simulink model "mfordmodel_v1"  (R2023a)
settings: Solver=ode45  StartTime=0.0  StopTime=10.0  RelTol=1e-3  EnableMultiTasking=on
undefined symbols (not defined in the file): ABV_RATIO_SW, AC_OFF_DLY, ACLOD, AUTO_TRNS_SW, BRAKE_DNDT_X, BZZRPM, BZZRPM_ALT, BZZTM, BZZTM_ALT, CMD_LITOFF, CMD_STABLE, CO_ST_ECT__A, COOL_BASE, DAS_BKDLY_A, DAS_CNT, DAS_CTDLY, DAS_LC_SW__A, DASCLP_5INH, DASCTL, DASMHYST, DASMPH, DEBYCP, DES_BASE, DPNEU_MUL, DSDRPM_DN_TC, DSDRPM_OFF, DSDRPM_UP_TC, EDF_DELAY, EDFHP, ETC_CL_TP, ETC_HP, GR_CM_CREEP, HCAM_ACT_CLP, HEDFHP, HEDFRPM, HICAM_PS, IAC_CAL_SW, IAC_ER_TM1, IAC_ER_TM2, IAC_ER_TM4, IAC_HI_LIM__A, IAC_ISFL_OBD, IAC_KAM_SW, IAC_LO_LIM__A, IAC_MON_TM, IAC_OT_REQ, IAC_RUN_TM, IAC_TP_OBD, IAC_TR_DAS, IAC_TST_DC, ID_DAS__A, ID_NOVS__A, IDVS_CH__A, IDVS_SL__A, IPSI_SW, IPSIDLY, IS_DRBASE__A, IS_DRBASE_A__A, IS_NUBASE__A, IS_NUBASE_A__A ... (+35)
libraries: simulink x2
(part 4 of 12)

== system mfordmodel_v1/iac_v04_001_001/iac_executive/mode_control/external_override_mode ==
  trig_external_override_mode : Inport
  osm_eo_off : Inport  Port=2
  osm_eo_on : Inport  Port=3
  osc_ena_0 : Inport  Port=4
  osc_state : Inport  Port=5
  abv_flowrate_in : Inport  Port=6
  abv_ratio_in : Inport  Port=7
  external_override_mode_ctl : Stateflow chart  TreatAsAtomicUnit=on
  flowrate_set : Subsystem  TreatAsAtomicUnit=on  mask(flowrate_set){}
      mask help: TBD
      mask Display:
      | disp('\n
      | IF (ml_flow_sel_sw == 1) THEN           \n
      |  substitute(0, abv_flowrate)\n
      | abv_ratio = 0.0                   \n
      | ELSE IF (ml_flow_sel_sw == 2) THEN\n
      | abv_flowrate = 15.99976    \n
      | abv_ratio = 0.0                    \n
      | ELSE IF (ml_flow_sel_sw == 3) THEN\n
      | abv_flowrate = 0.0              \n
      | abv_ratio = 0.0                   \n
      | ELSE IF (ml_flow_sel_sw == 4) THEN\n
      |     Do Nothing;                      \n
      | ENDIF                                                ')
  substitute : Subsystem  TreatAsAtomicUnit=on  mask(substitute){channel=0}
      mask prompts: channel "Select OSC channel"
      mask help: This block will perform Output State Control (OSC) substitution, for now it is strictly a pass-through block.
      mask TypeOptions channel: 0 | 1 | 2 | 3 | 4 | 5 | 6 | 7 | 8 | 9 | 10 | 11 | 12 | 15 | 16 | 17 | 18 | 19 | 20 | 21 | 22 | 23 | 24 | 25 | 26 | 27 | 28 | 29 | 30 | 31 | 32 | 33 | 34 | 35 | 36 | 37 | 38 | 39 | 40 | 41 | 42 | 43 | 44 | 45 | 46 | 47 | 48 | 49 | 50
      mask Display: fprintf('\nChannel # = %s\n',channel);
  abv_flowrate : Outport
  abv_ratio : Outport  Port=2
  wires:
  abv_ratio_in/1 -> flowrate_set/4(abv_ratio_in)
  flowrate_set/2(abv_ratio) -> abv_ratio/1
  flowrate_set/1(abv_flowrate) -> abv_flowrate/1
  abv_flowrate_in/1 -> flowrate_set/3(abv_flowrate_in), substitute/1(OSC_in)
  substitute/1(OSC_out) -> flowrate_set/2(abv_flowrate_osc)  "abv_flowrate_osc"
  external_override_mode_ctl/2(do_flowrate_set()) -> flowrate_set/Trigger  "do_flowrate_set"
  external_override_mode_ctl/1(ml_flow_sel_sw) -> flowrate_set/1(ml_flow_sel_sw)  "ml_flow_sel_sw"
  external_override_mode_ctl/3(do_substitute()) -> substitute/Trigger  "do_substitute"
  osc_ena_0/1 -> external_override_mode_ctl/3(osc_ena_0)
  osc_state/1 -> external_override_mode_ctl/4(osc_state)
  osm_eo_off/1 -> external_override_mode_ctl/1(osm_eo_off)
  osm_eo_on/1 -> external_override_mode_ctl/2(osm_eo_on)
  trig_external_override_mode/1 -> external_override_mode_ctl/Trigger

== system mfordmodel_v1/iac_v04_001_001/iac_executive/mode_control/failure_mode ==
  do_failure_mode : TriggerPort  TriggerType=function-call  VariantControl=(inherit)
  CONSTANT1 : Subsystem  mask(Constant){constant=IAC_FM_PPM}
      mask help: Constant Block. Will dispaly constant name and value on the icon of the block
      mask init:
      | if isletter(constant(1))
      |   const = evalin('base',constant);
      |   name = constant;
      | else
      |   const = str2num(constant);
      |   name = 'CONST';
      | end;
      mask Display: fprintf('%s = %.4f',name,const);
  Constant1 : Constant  Value=0
  Constant2 : Constant
  ISCFLG_DASHPOT_PREPOSITION : Constant  Value=0
  abv_flowrate : Outport  InitialOutput=[0]
  abv_ratio : Outport  Port=2  InitialOutput=[0]
  hcamfg : Outport  Port=3  InitialOutput=[0]
  iscflg : Outport  Port=4  InitialOutput=[0]
  wires:
  ISCFLG_DASHPOT_PREPOSITION/1 -> iscflg/1  "iscflg"
  CONSTANT1/1(Out) -> abv_flowrate/1  "abv_flowrate"
  Constant1/1 -> abv_ratio/1  "abv_ratio"
  Constant2/1 -> hcamfg/1  "hcamfg"

== system mfordmodel_v1/iac_v04_001_001/iac_executive/runup_flag_timer/TIMER_DT_in ==
  note: timer14/TIMER
  note: Timer Control calls functions within the Time Calculator
      | after using the flags 'increment_flag' and 'decrement_flag'
      | to determine the direction of the timer.
  trig_time : Inport
  trig_reset : Inport  Port=2
  reset value : Inport  Port=3
  inc flag : Inport  Port=4
  dec flag : Inport  Port=5
  delta time : Inport  Port=6
  Event Triggers : Mux  Inputs=2
  Time Calculator : Subsystem
  Timer Control : Stateflow chart  TreatAsAtomicUnit=on
  timer : Outport
  wires:
  inc flag/1 -> Timer Control/1(incr_flag)  "increment_flag"
  dec flag/1 -> Timer Control/2(decr_flag)  "decrement_flag"
  Timer Control/4(do_timer()) -> Time Calculator/4(do_timer)  "do_timer"
  Timer Control/3(do_delta_time()) -> Time Calculator/3(do_delta_time)  "do_delta_time"
  Timer Control/2(reset_flag) -> Time Calculator/2(reset_val)  "reset_flag"
  Timer Control/1(count_direction) -> Time Calculator/1(count_direction)  "count_direction"
  Time Calculator/1(timer) -> timer/1  "timer"
  Event Triggers/1 -> Timer Control/Trigger
  trig_time/1 -> Event Triggers/1  "trig_timer"
  trig_reset/1 -> Event Triggers/2  "trig_reset"
  reset value/1 -> Time Calculator/5(reset_value)  "reset_value"
  delta time/1 -> Time Calculator/6(delta time)  "delta_time"

== system mfordmodel_v1/iac_v04_001_001/normal_mode/activate_feedforward/ac_ppm_tmr ==
  note: Timer Control calls functions within the Time Calculator
      | after using the flags 'increment_flag' and 'decrement_flag'
      | to determine the direction of the timer.
  note: timer14/TIMER
  trig_time : Inport
  trig_reset : Inport  Port=2
  reset value : Inport  Port=3
  inc flag : Inport  Port=4
  dec flag : Inport  Port=5
  Event Triggers : Mux  Inputs=2
  Time Calculator : Subsystem
  Timer Control : Stateflow chart  TreatAsAtomicUnit=on
  timer : Outport
  wires:
  reset value/1 -> Time Calculator/5(reset_value)  "reset_value"
  trig_reset/1 -> Event Triggers/2  "trig_reset"
  trig_time/1 -> Event Triggers/1  "trig_timer"
  Event Triggers/1 -> Timer Control/Trigger
  Time Calculator/1(timer) -> timer/1  "timer"
  Timer Control/1(count_direction) -> Time Calculator/1(count_direction)  "count_direction"
  Timer Control/2(reset_flag) -> Time Calculator/2(reset_val)  "reset_flag"
  Timer Control/3(do_delta_time()) -> Time Calculator/3(do_delta_time)  "do_delta_time"
  Timer Control/4(do_timer()) -> Time Calculator/4(do_timer)  "do_timer"
  dec flag/1 -> Timer Control/2(decr_flag)  "decrement_flag"
  inc flag/1 -> Timer Control/1(incr_flag)  "increment_flag"

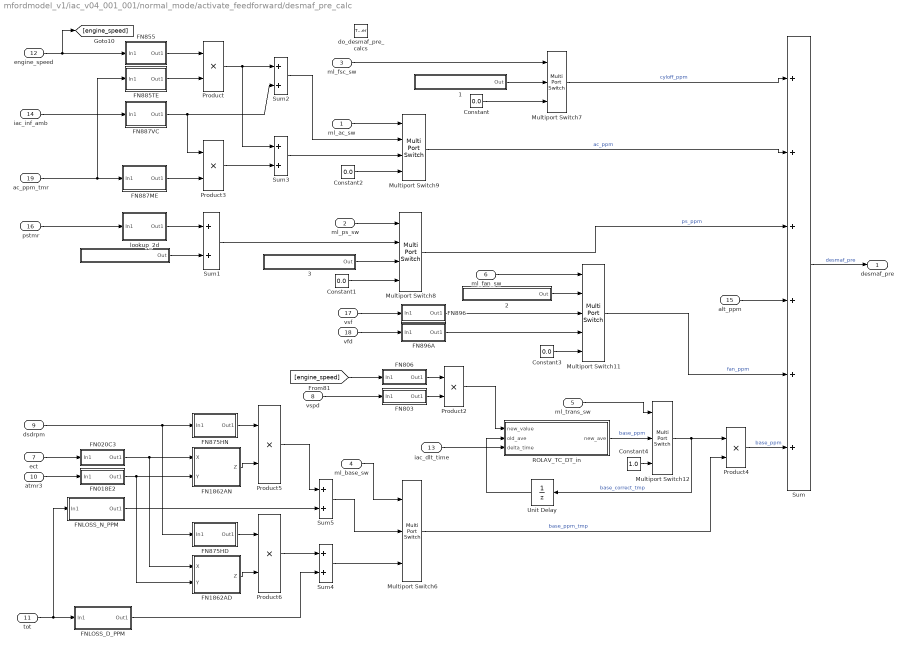
== system mfordmodel_v1/iac_v04_001_001/normal_mode/activate_feedforward/desmaf_pre_calc ==
  ml_ac_sw : Inport
  ml_ps_sw : Inport  Port=2
  ml_fsc_sw : Inport  Port=3
  ml_base_sw : Inport  Port=4
  ml_trans_sw : Inport  Port=5
  ml_fan_sw : Inport  Port=6
  ect : Inport  Port=7
  vspd : Inport  Port=8
  dsdrpm : Inport  Port=9
  atmr3 : Inport  Port=10
  tot : Inport  Port=11
  engine_speed : Inport  Port=12
  iac_dlt_time : Inport  Port=13
  iac_inf_amb : Inport  Port=14
  alt_ppm : Inport  Port=15
  pstmr : Inport  Port=16
  vsf : Inport  Port=17
  vfd : Inport  Port=18
  ac_ppm_tmr : Inport  Port=19
  do_desmaf_pre_calcs : TriggerPort  TriggerType=function-call  VariantControl=(inherit)
  "  " : Subsystem  mask(Constant){constant=PSPPM}
      mask help: Constant Block. Will dispaly constant name and value on the icon of the block
      mask init:
      | if isletter(constant(1))
      |   const = evalin('base',constant);
      |   name = constant;
      | else
      |   const = str2num(constant);
      |   name = 'CONST';
      | end;
      mask Display: fprintf('%s = %.4f',name,const);
  "  2" : Subsystem  mask(Constant){constant=EDFPPM}
      mask help: Constant Block. Will dispaly constant name and value on the icon of the block
      mask init:
      | if isletter(constant(1))
      |   const = evalin('base',constant);
      |   name = constant;
      | else
      |   const = str2num(constant);
      |   name = 'CONST';
      | end;
      mask Display: fprintf('%s = %.4f',name,const);
  1 : Subsystem  mask(Constant){constant=FSC_BASE_PPM}
      mask help: Constant Block. Will dispaly constant name and value on the icon of the block
      mask init:
      | if isletter(constant(1))
      |   const = evalin('base',constant);
      |   name = constant;
      | else
      |   const = str2num(constant);
      |   name = 'CONST';
      | end;
      mask Display: fprintf('%s = %.4f',name,const);
  3 : Subsystem  mask(Constant){constant=PSPPM_VS}
      mask help: Constant Block. Will dispaly constant name and value on the icon of the block
      mask init:
      | if isletter(constant(1))
      |   const = evalin('base',constant);
      |   name = constant;
      | else
      |   const = str2num(constant);
      |   name = 'CONST';
      | end;
      mask Display: fprintf('%s = %.4f',name,const);
  Constant{,1..3} (4 alike) : Constant  Value=0.0
  Constant4 : Constant  Value=1.0
  FN018E2 : Subsystem  mask(2-D, piece-wise, linear interpolation){CAL_FUNC=FN018E}
      mask prompts: CAL_FUNC "Calibration function name"
      mask help:
      | Performs piece-wise linear interpolation.
      |
      | Output is NOT extrapolated beyond the input range.  If the input value presented to the block lies outside the range specified in the block's parameter, then the value is treated as though it has the value of the nearest value in the range.
      mask init: same as mfordmodel_v1/iac_v04_001_001/activate_desired_rpm/rpm_calcs/lookup_2d
      mask Help:
      | Enter the name of the calibration function.
      | (e.g. EGM_VA_ECT_MULT)
      mask Display:
      | fprintf('%s',CAL_FUNC);
      | plot(calfunc.X,calfunc.Y,max_x*1.05,max_y*1.05,min_x,min_y);
  FN020C3 : Subsystem  mask(2-D, piece-wise, linear interpolation){CAL_FUNC=FN020C}
      mask prompts: CAL_FUNC "Calibration function name"
      mask help:
      | Performs piece-wise linear interpolation.
      |
      | Output is NOT extrapolated beyond the input range.  If the input value presented to the block lies outside the range specified in the block's parameter, then the value is treated as though it has the value of the nearest value in the range.
      mask init: same as mfordmodel_v1/iac_v04_001_001/activate_desired_rpm/rpm_calcs/lookup_2d
      mask Help:
      | Enter the name of the calibration function.
      | (e.g. EGM_VA_ECT_MULT)
      mask Display:
      | fprintf('%s',CAL_FUNC);
      | plot(calfunc.X,calfunc.Y,max_x*1.05,max_y*1.05,min_x,min_y);
  FN1862AD : Subsystem  mask(3-D, piece-wise, linear interpolation){CAL_TABLE=FN1862AD}
      mask prompts: CAL_TABLE "Calibration table name"
      mask help:
      | Performs 3-D, piece-wise linear interpolation.
      |
      | Output is NOT extrapolated beyond the input ranges.  If an input value presented to the block lies outside the range specified in the block's parameters, then the value is treated as though it has the value of the nearest value in the range.
      mask init:
      | if isempty(CAL_TABLE) |  isspace(CAL_TABLE)
      |  caltable.Z=[0 .05 .1 .1 ;.1 .15 .2 .2; .2 .25 .3 .3;.3 .35 .4 .4];
      |  min_x=0;
      |  min_y=0;
      |  max_x=3;
      |  max_y=3;
      |  minz=0;
      |  maxz=1;
      |  CAL_TABLE='FNxxxx';
      | else
      |   caltable = evalin('base',CAL_TABLE);
      |   min_x = caltable.X(1);
      |   max_x = caltable.X(length(caltable.X));
      |   min_y = caltable.Y(1);
      |   max_y = caltable.Y(length(caltable.Y));
      |   minz=min(min(caltable.Z));
      |   maxz=max(max(caltable.Z));
      | end
      mask Help: Enter the name of the calibration table.
      mask Display:
      | fprintf('%s',CAL_TABLE);
      | plot(caltable.Z');
      | plot([min_x max_x],[minz*.99 minz*.99]);
      | plot([min_x min_x],[minz*.99 maxz*1.01]);
  FN1862AN : Subsystem  mask(3-D, piece-wise, linear interpolation){CAL_TABLE=FN1862AN}
      mask prompts: CAL_TABLE "Calibration table name"
      mask help:
      | Performs 3-D, piece-wise linear interpolation.
      |
      | Output is NOT extrapolated beyond the input ranges.  If an input value presented to the block lies outside the range specified in the block's parameters, then the value is treated as though it has the value of the nearest value in the range.
      mask init: same as mfordmodel_v1/iac_v04_001_001/normal_mode/activate_feedforward/desmaf_pre_calc/FN1862AD
      mask Help: Enter the name of the calibration table.
      mask Display:
      | fprintf('%s',CAL_TABLE);
      | plot(caltable.Z');
      | plot([min_x max_x],[minz*.99 minz*.99]);
      | plot([min_x min_x],[minz*.99 maxz*1.01]);
  FN803 : Subsystem  mask(2-D, piece-wise, linear interpolation){CAL_FUNC=FN802}
      mask prompts: CAL_FUNC "Calibration function name"
      mask help:
      | Performs piece-wise linear interpolation.
      |
      | Output is NOT extrapolated beyond the input range.  If the input value presented to the block lies outside the range specified in the block's parameter, then the value is treated as though it has the value of the nearest value in the range.
      mask init: same as mfordmodel_v1/iac_v04_001_001/activate_desired_rpm/rpm_calcs/lookup_2d
      mask Help:
      | Enter the name of the calibration function.
      | (e.g. EGM_VA_ECT_MULT)
      mask Display:
      | fprintf('%s',CAL_FUNC);
      | plot(calfunc.X,calfunc.Y,max_x*1.05,max_y*1.05,min_x,min_y);
  FN806 : Subsystem  mask(2-D, piece-wise, linear interpolation){CAL_FUNC=FN805}
      mask prompts: CAL_FUNC "Calibration function name"
      mask help:
      | Performs piece-wise linear interpolation.
      |
      | Output is NOT extrapolated beyond the input range.  If the input value presented to the block lies outside the range specified in the block's parameter, then the value is treated as though it has the value of the nearest value in the range.
      mask init: same as mfordmodel_v1/iac_v04_001_001/activate_desired_rpm/rpm_calcs/lookup_2d
      mask Help:
      | Enter the name of the calibration function.
      | (e.g. EGM_VA_ECT_MULT)
      mask Display:
      | fprintf('%s',CAL_FUNC);
      | plot(calfunc.X,calfunc.Y,max_x*1.05,max_y*1.05,min_x,min_y);
  FN855 : Subsystem  mask(2-D, piece-wise, linear interpolation){CAL_FUNC=FN885}
      mask prompts: CAL_FUNC "Calibration function name"
      mask help:
      | Performs piece-wise linear interpolation.
      |
      | Output is NOT extrapolated beyond the input range.  If the input value presented to the block lies outside the range specified in the block's parameter, then the value is treated as though it has the value of the nearest value in the range.
      mask init: same as mfordmodel_v1/iac_v04_001_001/activate_desired_rpm/rpm_calcs/lookup_2d
      mask Help:
      | Enter the name of the calibration function.
      | (e.g. EGM_VA_ECT_MULT)
      mask Display:
      | fprintf('%s',CAL_FUNC);
      | plot(calfunc.X,calfunc.Y,max_x*1.05,max_y*1.05,min_x,min_y);
  FN875HD : Subsystem  mask(2-D, piece-wise, linear interpolation){CAL_FUNC=FN875HD}
      mask prompts: CAL_FUNC "Calibration function name"
      mask help:
      | Performs piece-wise linear interpolation.
      |
      | Output is NOT extrapolated beyond the input range.  If the input value presented to the block lies outside the range specified in the block's parameter, then the value is treated as though it has the value of the nearest value in the range.
      mask init: same as mfordmodel_v1/iac_v04_001_001/activate_desired_rpm/rpm_calcs/lookup_2d
      mask Help:
      | Enter the name of the calibration function.
      | (e.g. EGM_VA_ECT_MULT)
      mask Display:
      | fprintf('%s',CAL_FUNC);
      | plot(calfunc.X,calfunc.Y,max_x*1.05,max_y*1.05,min_x,min_y);
  FN875HN : Subsystem  mask(2-D, piece-wise, linear interpolation){CAL_FUNC=FN875HN}
      mask prompts: CAL_FUNC "Calibration function name"
      mask help:
      | Performs piece-wise linear interpolation.
      |
      | Output is NOT extrapolated beyond the input range.  If the input value presented to the block lies outside the range specified in the block's parameter, then the value is treated as though it has the value of the nearest value in the range.
      mask init: same as mfordmodel_v1/iac_v04_001_001/activate_desired_rpm/rpm_calcs/lookup_2d
      mask Help:
      | Enter the name of the calibration function.
      | (e.g. EGM_VA_ECT_MULT)
      mask Display:
      | fprintf('%s',CAL_FUNC);
      | plot(calfunc.X,calfunc.Y,max_x*1.05,max_y*1.05,min_x,min_y);
  FN885TE : Subsystem  mask(2-D, piece-wise, linear interpolation){CAL_FUNC=FN885TE}
      mask prompts: CAL_FUNC "Calibration function name"
      mask help:
      | Performs piece-wise linear interpolation.
      |
      | Output is NOT extrapolated beyond the input range.  If the input value presented to the block lies outside the range specified in the block's parameter, then the value is treated as though it has the value of the nearest value in the range.
      mask init: same as mfordmodel_v1/iac_v04_001_001/activate_desired_rpm/rpm_calcs/lookup_2d
      mask Help:
      | Enter the name of the calibration function.
      | (e.g. EGM_VA_ECT_MULT)
      mask Display:
      | fprintf('%s',CAL_FUNC);
      | plot(calfunc.X,calfunc.Y,max_x*1.05,max_y*1.05,min_x,min_y);
  FN887ME : Subsystem  mask(2-D, piece-wise, linear interpolation){CAL_FUNC=FN887ME}
      mask prompts: CAL_FUNC "Calibration function name"
      mask help:
      | Performs piece-wise linear interpolation.
      |
      | Output is NOT extrapolated beyond the input range.  If the input value presented to the block lies outside the range specified in the block's parameter, then the value is treated as though it has the value of the nearest value in the range.
      mask init: same as mfordmodel_v1/iac_v04_001_001/activate_desired_rpm/rpm_calcs/lookup_2d
      mask Help:
      | Enter the name of the calibration function.
      | (e.g. EGM_VA_ECT_MULT)
      mask Display:
      | fprintf('%s',CAL_FUNC);
      | plot(calfunc.X,calfunc.Y,max_x*1.05,max_y*1.05,min_x,min_y);
  FN887VC : Subsystem  mask(2-D, piece-wise, linear interpolation){CAL_FUNC=FN887VC}
      mask prompts: CAL_FUNC "Calibration function name"
      mask help:
      | Performs piece-wise linear interpolation.
      |
      | Output is NOT extrapolated beyond the input range.  If the input value presented to the block lies outside the range specified in the block's parameter, then the value is treated as though it has the value of the nearest value in the range.
      mask init: same as mfordmodel_v1/iac_v04_001_001/activate_desired_rpm/rpm_calcs/lookup_2d
      mask Help:
      | Enter the name of the calibration function.
      | (e.g. EGM_VA_ECT_MULT)
      mask Display:
      | fprintf('%s',CAL_FUNC);
      | plot(calfunc.X,calfunc.Y,max_x*1.05,max_y*1.05,min_x,min_y);
  FN896 : Subsystem  mask(2-D, piece-wise, linear interpolation){CAL_FUNC=FN896}
      mask prompts: CAL_FUNC "Calibration function name"
      mask help:
      | Performs piece-wise linear interpolation.
      |
      | Output is NOT extrapolated beyond the input range.  If the input value presented to the block lies outside the range specified in the block's parameter, then the value is treated as though it has the value of the nearest value in the range.
      mask init: same as mfordmodel_v1/iac_v04_001_001/activate_desired_rpm/rpm_calcs/lookup_2d
      mask Help:
      | Enter the name of the calibration function.
      | (e.g. EGM_VA_ECT_MULT)
      mask Display:
      | fprintf('%s',CAL_FUNC);
      | plot(calfunc.X,calfunc.Y,max_x*1.05,max_y*1.05,min_x,min_y);
  FN896A : Subsystem  mask(2-D, piece-wise, linear interpolation){CAL_FUNC=FN896A}
      mask prompts: CAL_FUNC "Calibration function name"
      mask help:
      | Performs piece-wise linear interpolation.
      |
      | Output is NOT extrapolated beyond the input range.  If the input value presented to the block lies outside the range specified in the block's parameter, then the value is treated as though it has the value of the nearest value in the range.
      mask init: same as mfordmodel_v1/iac_v04_001_001/activate_desired_rpm/rpm_calcs/lookup_2d
      mask Help:
      | Enter the name of the calibration function.
      | (e.g. EGM_VA_ECT_MULT)
      mask Display:
      | fprintf('%s',CAL_FUNC);
      | plot(calfunc.X,calfunc.Y,max_x*1.05,max_y*1.05,min_x,min_y);
  FNLOSS_D_PPM : Subsystem  mask(2-D, piece-wise, linear interpolation){CAL_FUNC=FNLOSS_D_PPM}
      mask prompts: CAL_FUNC "Calibration function name"
      mask help:
      | Performs piece-wise linear interpolation.
      |
      | Output is NOT extrapolated beyond the input range.  If the input value presented to the block lies outside the range specified in the block's parameter, then the value is treated as though it has the value of the nearest value in the range.
      mask init: same as mfordmodel_v1/iac_v04_001_001/activate_desired_rpm/rpm_calcs/lookup_2d
      mask Help:
      | Enter the name of the calibration function.
      | (e.g. EGM_VA_ECT_MULT)
      mask Display:
      | fprintf('%s',CAL_FUNC);
      | plot(calfunc.X,calfunc.Y,max_x*1.05,max_y*1.05,min_x,min_y);
  FNLOSS_N_PPM : Subsystem  mask(2-D, piece-wise, linear interpolation){CAL_FUNC=FNLOSS_N_PPM}
      mask prompts: CAL_FUNC "Calibration function name"
      mask help:
      | Performs piece-wise linear interpolation.
      |
      | Output is NOT extrapolated beyond the input range.  If the input value presented to the block lies outside the range specified in the block's parameter, then the value is treated as though it has the value of the nearest value in the range.
      mask init: same as mfordmodel_v1/iac_v04_001_001/activate_desired_rpm/rpm_calcs/lookup_2d
      mask Help:
      | Enter the name of the calibration function.
      | (e.g. EGM_VA_ECT_MULT)
      mask Display:
      | fprintf('%s',CAL_FUNC);
      | plot(calfunc.X,calfunc.Y,max_x*1.05,max_y*1.05,min_x,min_y);
  Multiport Switch11 : MultiPortSwitch  Inputs=4
  Multiport Switch12 : MultiPortSwitch  Inputs=2
  Multiport Switch6 : MultiPortSwitch  Inputs=2
  Multiport Switch7 : MultiPortSwitch  Inputs=2
  Multiport Switch8 : MultiPortSwitch
  Multiport Switch9 : MultiPortSwitch
  Product{,2..6} (6 alike) : Product  InputSameDT=on  RndMeth=Zero  SaturateOnIntegerOverflow=on  OutDataTypeStr=Inherit: Same as first input
  ROLAV_TC_DT_in : Subsystem  mask(Rolling Average - Time Constant){TAU=TCDAIR}
      mask prompts: TAU "Time Constant"
      mask help: Rolling Average - Time Constant. This filter block is the first order approximation using a time constant. Inputs include the time constant (entered through this dialogue), old_ave which is the previous average value, new_value which is the new filter to filter toward, and the delta_time which is elapsed time over which to perform the filter equation.
      mask init:
      | if isletter(TAU(1))
      |   tc = evalin('base',TAU);
      |   name = TAU;
      | else
      |   tc = str2num(TAU);
      |   name = 'TC';
      | end;
      mask Display: fprintf('%s = %.4f',name,tc);
  Sum : Sum  Inputs=++++++  InputSameDT=on  SaturateOnIntegerOverflow=on  OutDataTypeStr=Inherit: Same as first input
  Sum{1..5} (5 alike) : Sum  InputSameDT=on  SaturateOnIntegerOverflow=on  OutDataTypeStr=Inherit: Same as first input
  Unit Delay : UnitDelay  InitialCondition=1.0  SampleTime=-1
  lookup_2d : Subsystem  mask(2-D, piece-wise, linear interpolation){CAL_FUNC=FN822}
      mask prompts: CAL_FUNC "Calibration function name"
      mask help:
      | Performs piece-wise linear interpolation.
      |
      | Output is NOT extrapolated beyond the input range.  If the input value presented to the block lies outside the range specified in the block's parameter, then the value is treated as though it has the value of the nearest value in the range.
      mask init: same as mfordmodel_v1/iac_v04_001_001/activate_desired_rpm/rpm_calcs/lookup_2d
      mask Help:
      | Enter the name of the calibration function.
      | (e.g. EGM_VA_ECT_MULT)
      mask Display:
      | fprintf('%s',CAL_FUNC);
      | plot(calfunc.X,calfunc.Y,max_x*1.05,max_y*1.05,min_x,min_y);
  desmaf_pre : Outport
  wires:
  FN803/1(Out1) -> Product2/2
  FN806/1(Out1) -> Product2/1
  vspd/1 -> FN803/1(In1)
  [engine_speed] -> FN806/1(In1)
  Unit Delay/1 -> ROLAV_TC_DT_in/2(old_ave)
  Product2/1 -> ROLAV_TC_DT_in/1(new_value)
  iac_dlt_time/1 -> ROLAV_TC_DT_in/3(delta_time)
  Constant3/1 -> Multiport Switch11/5
  vfd/1 -> FN896A/1(In1)
  vsf/1 -> FN896/1(In1)
  FN896/1(Out1) -> Multiport Switch11/3
  Multiport Switch11/1 -> Sum/5  "fan_ppm"
  FN896A/1(Out1) -> Multiport Switch11/4
  "  2"/1(Out) -> Multiport Switch11/2
  ml_fan_sw/1 -> Multiport Switch11/1
  Multiport Switch12/1 -> Unit Delay/1, Product4/1  "base_correct_tmp"
  ROLAV_TC_DT_in/1(new_ave) -> Multiport Switch12/2  "base_ppm"
  ml_trans_sw/1 -> Multiport Switch12/1
  Constant4/1 -> Multiport Switch12/3
  Multiport Switch6/1 -> Product4/2  "base_ppm_tmp"
  FN875HN/1(Out1) -> Product5/1
  FN1862AN/1(Z) -> Product5/2
  ml_base_sw/1 -> Multiport Switch6/1
  atmr3/1 -> FN018E2/1(In1)
  FN020C3/1(Out1) -> FN1862AN/1(X), FN1862AD/1(X)
  FN018E2/1(Out1) -> FN1862AN/2(Y), FN1862AD/2(Y)
  ect/1 -> FN020C3/1(In1)
  dsdrpm/1 -> FN875HN/1(In1), FN875HD/1(In1)
  Product5/1 -> Sum5/1
  FNLOSS_N_PPM/1(Out1) -> Sum5/2
  Sum5/1 -> Multiport Switch6/2
  Product6/1 -> Sum4/1
  Sum4/1 -> Multiport Switch6/3
  FNLOSS_D_PPM/1(Out1) -> Sum4/2
  FN875HD/1(Out1) -> Product6/1
  FN1862AD/1(Z) -> Product6/2
  tot/1 -> FNLOSS_D_PPM/1(In1), FNLOSS_N_PPM/1(In1)
  Product4/1 -> Sum/6  "base_ppm"
  Sum/1 -> desmaf_pre/1  "desmaf_pre"
  FN855/1(Out1) -> Product/1
  FN885TE/1(Out1) -> Product/2
  alt_ppm/1 -> Sum/4
  Multiport Switch8/1 -> Sum/3  "ps_ppm"
  Multiport Switch9/1 -> Sum/2  "ac_ppm"
  Sum2/1 -> Multiport Switch9/2
  Sum3/1 -> Multiport Switch9/3
  Constant2/1 -> Multiport Switch9/4
  ml_ac_sw/1 -> Multiport Switch9/1
  Product3/1 -> Sum3/2
  FN887ME/1(Out1) -> Product3/2
  Product/1 -> Sum2/1, Sum3/1
  FN887VC/1(Out1) -> Sum2/2, Product3/1
  engine_speed/1 -> [engine_speed], FN855/1(In1)
  iac_inf_amb/1 -> FN887VC/1(In1)
  ac_ppm_tmr/1 -> FN887ME/1(In1), FN885TE/1(In1)
  lookup_2d/1(Out1) -> Sum1/1
  "  "/1(Out) -> Sum1/2
  Constant1/1 -> Multiport Switch8/4
  ml_ps_sw/1 -> Multiport Switch8/1
  3/1(Out) -> Multiport Switch8/3
  Sum1/1 -> Multiport Switch8/2
  pstmr/1 -> lookup_2d/1(In1)
  Multiport Switch7/1 -> Sum/1  "cyloff_ppm"
  Constant/1 -> Multiport Switch7/3
  1/1(Out) -> Multiport Switch7/2
  ml_fsc_sw/1 -> Multiport Switch7/1

== system mfordmodel_v1/iac_v04_001_001/normal_mode/activate_kam/iac_kam_tmr ==
  note: Timer Control calls functions within the Time Calculator
      | after using the flags 'increment_flag' and 'decrement_flag'
      | to determine the direction of the timer.
  note: timer14/TIMER
  trig_time : Inport
  trig_reset : Inport  Port=2
  reset value : Inport  Port=3
  inc flag : Inport  Port=4
  dec flag : Inport  Port=5
  Event Triggers : Mux  Inputs=2
  Time Calculator : Subsystem
  Timer Control : Stateflow chart  TreatAsAtomicUnit=on
  timer : Outport
  wires:
  reset value/1 -> Time Calculator/5(reset_value)  "reset_value"
  trig_reset/1 -> Event Triggers/2  "trig_reset"
  trig_time/1 -> Event Triggers/1  "trig_timer"
  Event Triggers/1 -> Timer Control/Trigger
  Time Calculator/1(timer) -> timer/1  "timer"
  Timer Control/1(count_direction) -> Time Calculator/1(count_direction)  "count_direction"
  Timer Control/2(reset_flag) -> Time Calculator/2(reset_val)  "reset_flag"
  Timer Control/3(do_delta_time()) -> Time Calculator/3(do_delta_time)  "do_delta_time"
  Timer Control/4(do_timer()) -> Time Calculator/4(do_timer)  "do_timer"
  dec flag/1 -> Timer Control/2(decr_flag)  "decrement_flag"
  inc flag/1 -> Timer Control/1(incr_flag)  "increment_flag"

== system mfordmodel_v1/iac_v04_001_001/normal_mode/activate_kam/isckam_calcs ==
  ipsibr_fb : Inport
  ml_kam_inc_sw : Inport  Port=2
  ml_isflag_sw : Inport  Port=3
  isckam_in : Inport  Port=4
  iac_ac_n_kam_in : Inport  Port=5
  iac_ac_d_kam_in : Inport  Port=6
  do_isckam_calcs : TriggerPort  TriggerType=function-call  VariantControl=(inherit)
  Bus Selector2 : BusSelector  OutputSignals=isckam0
  Bus Selector3 : BusSelector  OutputSignals=isckam2
  Constant1 : Constant  Value=0.0
  Constant7 : Constant  Value=.0003
  Constant8 : Constant  Value=-.0003
  Multiport Switch{17..18,24..25} (4 alike) : MultiPortSwitch  Inputs=4
  Multiport Switch23 : MultiPortSwitch
  Mux : Mux
  Sum{10..13} (4 alike) : Sum  Inputs=|++  InputSameDT=on  SaturateOnIntegerOverflow=on  OutDataTypeStr=Inherit: Same as first input
  Sum15 : Sum  Inputs=+-  InputSameDT=on  SaturateOnIntegerOverflow=on  OutDataTypeStr=Inherit: Same as first input
  Sum16 : Sum  InputSameDT=on  SaturateOnIntegerOverflow=on  OutDataTypeStr=Inherit: Same as first input
  Sum18 : Sum  InputSameDT=on  SaturateOnIntegerOverflow=on  OutDataTypeStr=Inherit: Same as first input
  ipsibr_kam : Outport
  isckam : Outport  Port=2
  iac_ac_n_kam : Outport  Port=3
  iac_ac_d_kam : Outport  Port=4
  wires:
  ml_kam_inc_sw/1 -> Multiport Switch23/1
  Constant1/1 -> Multiport Switch23/4
  Constant8/1 -> Multiport Switch23/2
  Constant7/1 -> Multiport Switch23/3
  Multiport Switch23/1 -> [increment_tmp], Sum15/2  "increment_tmp"
  Mux/1 -> isckam/1  "ml_isckam"
  Sum16/1 -> Mux/2  "isckam1"
  Sum18/1 -> Mux/4  "isckam3"
  [ml_isflag_sw] -> Multiport Switch18/1
  Sum11/1 -> Multiport Switch18/4
  [increment_tmp] -> Sum11/1
  Sum10/1 -> Multiport Switch17/5
  [ml_isflag_sw] -> Multiport Switch17/1
  [increment_tmp] -> Sum10/2
  [ml_isflag_sw] -> Multiport Switch24/1
  Sum12/1 -> Multiport Switch24/3
  [increment_tmp] -> Sum12/1
  ml_isflag_sw/1 -> [ml_isflag_sw], Multiport Switch25/1
  Sum13/1 -> Multiport Switch25/2
  [increment_tmp] -> Sum13/1
  isckam_in/1 -> Bus Selector2/1, Bus Selector3/1
  ipsibr_fb/1 -> Sum15/1
  Sum15/1 -> ipsibr_kam/1  "ipsibr_kam"
  Multiport Switch17/1 -> iac_ac_n_kam/1  "iac_ac_n_kam"
  iac_ac_n_kam_in/1 -> Multiport Switch17/2, Multiport Switch17/3, Multiport Switch17/4, Sum10/1, [iac_ac_n_kam]
  Multiport Switch24/1 -> iac_ac_d_kam/1  "iac_ac_d_kam"
  iac_ac_d_kam_in/1 -> Multiport Switch24/2, Multiport Switch24/5, Multiport Switch24/4, Sum12/2, [iac_ac_d_kam]
  Multiport Switch25/1 -> Mux/1  "isckam0"
  Multiport Switch18/1 -> Mux/3  "isckam2"
  Bus Selector2/1 -> Multiport Switch25/5, Sum13/2, Multiport Switch25/3, Multiport Switch25/4, [isckam0]  "<isckam0>"
  Bus Selector3/1 -> Multiport Switch18/2, Multiport Switch18/3, Multiport Switch18/5, Sum11/2, [isckam2]  "<isckam2>"
  [iac_ac_d_kam] -> Sum16/2
  [isckam0] -> Sum16/1
  [iac_ac_n_kam] -> Sum18/2
  [isckam2] -> Sum18/1

== system mfordmodel_v1/iac_v04_001_001/normal_mode/activate_kam/isckam_clear ==
  note: These connection is made via
      | a constant block here instead of a goto/from
      | tag because the actual signals
      | are connected to merge blocks and sumulink
      | does not allow multiple connections for
      | signal lines connected to merge blocks.
  do_isckam_clear : TriggerPort  TriggerType=function-call  VariantControl=(inherit)
  CONSTANT1 : Subsystem  mask(Constant){constant=IAC_AC_START}
      mask help: Constant Block. Will dispaly constant name and value on the icon of the block
      mask init:
      | if isletter(constant(1))
      |   const = evalin('base',constant);
      |   name = constant;
      | else
      |   const = str2num(constant);
      |   name = 'CONST';
      | end;
      mask Display: fprintf('%s = %.4f',name,const);
  CONSTANT2 : Subsystem  mask(Constant){constant=IAC_NU_START}
      mask help: Constant Block. Will dispaly constant name and value on the icon of the block
      mask init:
      | if isletter(constant(1))
      |   const = evalin('base',constant);
      |   name = constant;
      | else
      |   const = str2num(constant);
      |   name = 'CONST';
      | end;
      mask Display: fprintf('%s = %.4f',name,const);
  CONSTANT3 : Subsystem  mask(Constant){constant=IAC_DR_START}
      mask help: Constant Block. Will dispaly constant name and value on the icon of the block
      mask init:
      | if isletter(constant(1))
      |   const = evalin('base',constant);
      |   name = constant;
      | else
      |   const = str2num(constant);
      |   name = 'CONST';
      | end;
      mask Display: fprintf('%s = %.4f',name,const);
  CONSTANT4 : Subsystem  mask(Constant){constant=IAC_AC_START}
      mask help: Constant Block. Will dispaly constant name and value on the icon of the block
      mask init:
      | if isletter(constant(1))
      |   const = evalin('base',constant);
      |   name = constant;
      | else
      |   const = str2num(constant);
      |   name = 'CONST';
      | end;
      mask Display: fprintf('%s = %.4f',name,const);
  CONSTANT5 : Subsystem  mask(Constant){constant=IAC_DR_START}
      mask help: Constant Block. Will dispaly constant name and value on the icon of the block
      mask init:
      | if isletter(constant(1))
      |   const = evalin('base',constant);
      |   name = constant;
      | else
      |   const = str2num(constant);
      |   name = 'CONST';
      | end;
      mask Display: fprintf('%s = %.4f',name,const);
  CONSTANT6 : Subsystem  mask(Constant){constant=IAC_NU_START}
      mask help: Constant Block. Will dispaly constant name and value on the icon of the block
      mask init:
      | if isletter(constant(1))
      |   const = evalin('base',constant);
      |   name = constant;
      | else
      |   const = str2num(constant);
      |   name = 'CONST';
      | end;
      mask Display: fprintf('%s = %.4f',name,const);
  CONSTANT7 : Subsystem  mask(Constant){constant=IAC_AC_START}
      mask help: Constant Block. Will dispaly constant name and value on the icon of the block
      mask init:
      | if isletter(constant(1))
      |   const = evalin('base',constant);
      |   name = constant;
      | else
      |   const = str2num(constant);
      |   name = 'CONST';
      | end;
      mask Display: fprintf('%s = %.4f',name,const);
  CONSTANT8 : Subsystem  mask(Constant){constant=IAC_AC_START}
      mask help: Constant Block. Will dispaly constant name and value on the icon of the block
      mask init:
      | if isletter(constant(1))
      |   const = evalin('base',constant);
      |   name = constant;
      | else
      |   const = str2num(constant);
      |   name = 'CONST';
      | end;
      mask Display: fprintf('%s = %.4f',name,const);
  Constant : Constant  Value=0.0
  Constant1 : Constant  Value=0.0
  Mux : Mux
  Sum1 : Sum  Inputs=++++  InputSameDT=on  SaturateOnIntegerOverflow=on  OutDataTypeStr=Inherit: Same as first input
  isckam : Outport
  iac_ac_n_kam : Outport  Port=2
  iac_ac_d_kam : Outport  Port=3
  iac_chksum : Outport  Port=4
  wires:
  Mux/1 -> isckam/1  "ml_isckam"
  Constant/1 -> Mux/2  "isckam1"
  Constant1/1 -> Mux/4  "isckam3"
  CONSTANT3/1(Out) -> Mux/1  "isckam0"
  CONSTANT2/1(Out) -> Mux/3  "isckam2"
  Sum1/1 -> iac_chksum/1  "iac_chksum"
  CONSTANT5/1(Out) -> Sum1/2  "isckam0"
  CONSTANT6/1(Out) -> Sum1/1  "isckam2"
  CONSTANT7/1(Out) -> Sum1/3  "iac_ac_n_kam"
  CONSTANT8/1(Out) -> Sum1/4  "iac_ac_n_kam"
  CONSTANT1/1(Out) -> iac_ac_n_kam/1  "iac_ac_n_kam"
  CONSTANT4/1(Out) -> iac_ac_d_kam/1  "iac_ac_d_kam"

== system mfordmodel_v1/iac_v04_001_001/normal_mode/activate_kam/isckam_merge ==
  ml_isckam1 : Inport
  ml_isckam2 : Inport  Port=2
  Demux : Demux
      settings: DisplayOption=none
  Demux1 : Demux
      settings: DisplayOption=none
  Merge{3..6} (4 alike) : Merge
  Mux : Mux
  isckam : Outport
  wires:
  Demux1/4 -> Merge6/2
  Demux1/3 -> Merge5/2
  Demux1/2 -> Merge4/2
  Demux1/1 -> Merge3/2
  ml_isckam2/1 -> Demux1/1
  ml_isckam1/1 -> Demux/1
  Mux/1 -> isckam/1
  Merge6/1 -> Mux/4  "isckam3"
  Merge5/1 -> Mux/3  "isckam2"
  Merge4/1 -> Mux/2  "isckam1"
  Merge3/1 -> Mux/1  "isckam0"
  Demux/4 -> Merge6/1
  Demux/3 -> Merge5/1
  Demux/2 -> Merge4/1
  Demux/1 -> Merge3/1

== system mfordmodel_v1/iac_v04_001_001/normal_mode/activate_kam/isckam_update_checksum ==
  iac_ac_n_kam : Inport
  iac_ac_d_kam : Inport  Port=2
  isckam : Inport  Port=3
  do_isckam_update_checksum : TriggerPort  TriggerType=function-call  VariantControl=(inherit)
  Bus Selector3 : BusSelector  OutputSignals=isckam0,isckam2
  Sum7 : Sum  Inputs=++++  InputSameDT=on  SaturateOnIntegerOverflow=on  OutDataTypeStr=Inherit: Same as first input
  iac_chksum : Outport
  wires:
  isckam/1 -> Bus Selector3/1
  Bus Selector3/1 -> Sum7/3  "<isckam0>"
  Bus Selector3/2 -> Sum7/4  "<isckam2>"
  Sum7/1 -> iac_chksum/1  "iac_chksum"
  iac_ac_n_kam/1 -> Sum7/1
  iac_ac_d_kam/1 -> Sum7/2

== system mfordmodel_v1/iac_v04_001_001/normal_mode/activate_kam/kamsum_calc ==
  iac_ac_n_kam : Inport
  iac_ac_d_kam : Inport  Port=2
  isckam : Inport  Port=3
  iac_chksum : Inport  Port=4
  kamsum_calc : TriggerPort  TriggerType=function-call  VariantControl=(inherit)
  Abs : Abs
  Bus Selector2 : BusSelector  OutputSignals=isckam0,isckam2
  Sum6 : Sum  Inputs=++++-  InputSameDT=on  SaturateOnIntegerOverflow=on  OutDataTypeStr=Inherit: Same as first input
  ml_kamsum : Outport  InitialOutput=0
  wires:
  iac_chksum/1 -> Sum6/5
  Sum6/1 -> Abs/1
  isckam/1 -> Bus Selector2/1
  Bus Selector2/1 -> Sum6/3  "<isckam0>"
  Bus Selector2/2 -> Sum6/4  "<isckam2>"
  Abs/1 -> ml_kamsum/1  "ml_kamsum"
  iac_ac_n_kam/1 -> Sum6/1
  iac_ac_d_kam/1 -> Sum6/2

== system mfordmodel_v1/iac_v04_001_001/normal_mode/activate_kam/update_pids ==
  isckam : Inport
  do_update_pids : TriggerPort  TriggerType=function-call  VariantControl=(inherit)
  Bus Selector : BusSelector  OutputSignals=isckam0,isckam1,isckam2,isckam3
  CONSTANT1 : Subsystem  mask(Constant){constant=AUTO_TRNS_SW}
      mask help: Constant Block. Will dispaly constant name and value on the icon of the block
      mask init:
      | if isletter(constant(1))
      |   const = evalin('base',constant);
      |   name = constant;
      | else
      |   const = str2num(constant);
      |   name = 'CONST';
      | end;
      mask Display: fprintf('%s = %.4f',name,const);
  Constant9 : Constant  Value=0
  pid : Subsystem  mask(PID){pid_cat=J2190, pid_number=0x0976, bit=BIT_NONE}
      mask prompts: pid_cat "PID Category"; pid_number "PID Number (e.g., 0x0C or 0x1123)"
      mask help:
      | Generic PID - used for J1979 (modes 1,2) and J2190.
      |
      | PID number is either 2 (J1979) or 4 ( J2190) digits, preceeded by 0x.
      |
      | BIT is selected from a pop-up list.
      |
      | CTRL is either CTRL_NONE (default) or your control parameter which enables/disables reporting of the PID.
      mask TypeOptions pid_cat: J1979MODE1 | J1979MODE2 | J1979MODE6 | J2190
      mask TypeOptions bit: BIT_NONE | BIT_00 | BIT_01 | BIT_02 | BIT_03 | BIT_04 | BIT_05 | BIT_06 | BIT_07 | BIT_08 | BIT_09 | BIT_10 | BIT_11 | BIT_12 | BIT_13 | BIT_14 | BIT_15 | BIT_16 | BIT_17 | BIT_18 | BIT_19 | BIT_20 | BIT_21 | BIT_22 | BIT_23 | BIT_24 | BIT_25 | BIT_26 | BIT_27 | BIT_28 | BIT_29 | BIT_30 | BIT_31
      mask Display: fprintf('%s\n%s\n%s',pid_cat,pid_number,bit);
  pid1 : Subsystem  mask(PID){pid_cat=J2190, pid_number=0x0977, bit=BIT_NONE}
      mask prompts: pid_cat "PID Category"; pid_number "PID Number (e.g., 0x0C or 0x1123)"
      mask help:
      | Generic PID - used for J1979 (modes 1,2) and J2190.
      |
      | PID number is either 2 (J1979) or 4 ( J2190) digits, preceeded by 0x.
      |
      | BIT is selected from a pop-up list.
      |
      | CTRL is either CTRL_NONE (default) or your control parameter which enables/disables reporting of the PID.
      mask TypeOptions pid_cat: J1979MODE1 | J1979MODE2 | J1979MODE6 | J2190
      mask TypeOptions bit: BIT_NONE | BIT_00 | BIT_01 | BIT_02 | BIT_03 | BIT_04 | BIT_05 | BIT_06 | BIT_07 | BIT_08 | BIT_09 | BIT_10 | BIT_11 | BIT_12 | BIT_13 | BIT_14 | BIT_15 | BIT_16 | BIT_17 | BIT_18 | BIT_19 | BIT_20 | BIT_21 | BIT_22 | BIT_23 | BIT_24 | BIT_25 | BIT_26 | BIT_27 | BIT_28 | BIT_29 | BIT_30 | BIT_31
      mask Display: fprintf('%s\n%s\n%s',pid_cat,pid_number,bit);
  pid2 : Subsystem  mask(PID){pid_cat=J2190, pid_number=0x0978, bit=BIT_NONE}
      mask prompts: pid_cat "PID Category"; pid_number "PID Number (e.g., 0x0C or 0x1123)"
      mask help:
      | Generic PID - used for J1979 (modes 1,2) and J2190.
      |
      | PID number is either 2 (J1979) or 4 ( J2190) digits, preceeded by 0x.
      |
      | BIT is selected from a pop-up list.
      |
      | CTRL is either CTRL_NONE (default) or your control parameter which enables/disables reporting of the PID.
      mask TypeOptions pid_cat: J1979MODE1 | J1979MODE2 | J1979MODE6 | J2190
      mask TypeOptions bit: BIT_NONE | BIT_00 | BIT_01 | BIT_02 | BIT_03 | BIT_04 | BIT_05 | BIT_06 | BIT_07 | BIT_08 | BIT_09 | BIT_10 | BIT_11 | BIT_12 | BIT_13 | BIT_14 | BIT_15 | BIT_16 | BIT_17 | BIT_18 | BIT_19 | BIT_20 | BIT_21 | BIT_22 | BIT_23 | BIT_24 | BIT_25 | BIT_26 | BIT_27 | BIT_28 | BIT_29 | BIT_30 | BIT_31
      mask Display: fprintf('%s\n%s\n%s',pid_cat,pid_number,bit);
  pid3 : Subsystem  mask(PID){pid_cat=J2190, pid_number=0x0979, bit=BIT_NONE}
      mask prompts: pid_cat "PID Category"; pid_number "PID Number (e.g., 0x0C or 0x1123)"
      mask help:
      | Generic PID - used for J1979 (modes 1,2) and J2190.
      |
      | PID number is either 2 (J1979) or 4 ( J2190) digits, preceeded by 0x.
      |
      | BIT is selected from a pop-up list.
      |
      | CTRL is either CTRL_NONE (default) or your control parameter which enables/disables reporting of the PID.
      mask TypeOptions pid_cat: J1979MODE1 | J1979MODE2 | J1979MODE6 | J2190
      mask TypeOptions bit: BIT_NONE | BIT_00 | BIT_01 | BIT_02 | BIT_03 | BIT_04 | BIT_05 | BIT_06 | BIT_07 | BIT_08 | BIT_09 | BIT_10 | BIT_11 | BIT_12 | BIT_13 | BIT_14 | BIT_15 | BIT_16 | BIT_17 | BIT_18 | BIT_19 | BIT_20 | BIT_21 | BIT_22 | BIT_23 | BIT_24 | BIT_25 | BIT_26 | BIT_27 | BIT_28 | BIT_29 | BIT_30 | BIT_31
      mask Display: fprintf('%s\n%s\n%s',pid_cat,pid_number,bit);
  wires:
  CONSTANT1/1(Out) -> pid1/2(ctrl), pid/2(ctrl)
  isckam/1 -> Bus Selector/1
  Constant9/1 -> pid2/2(ctrl), pid3/2(ctrl)
  Bus Selector/1 -> pid/1(data)  "<isckam0>"
  Bus Selector/2 -> pid1/1(data)  "<isckam1>"
  Bus Selector/3 -> pid2/1(data)  "<isckam2>"
  Bus Selector/4 -> pid3/1(data)  "<isckam3>"

== system mfordmodel_v1/iac_v04_001_001/normal_mode/activate_normal_mode/dstpbr_calc ==
  ml_tc_sw : Inport
  tp : Inport  Port=2
  iac_dlt_time : Inport  Port=3
  dstpbr_in : Inport  Port=4
  do_dstpbr_calc : TriggerPort  TriggerType=function-call  VariantControl=(inherit)
  CONSTANT : Subsystem  mask(Constant){constant=TCDASU}
      mask help: Constant Block. Will dispaly constant name and value on the icon of the block
      mask init:
      | if isletter(constant(1))
      |   const = evalin('base',constant);
      |   name = constant;
      | else
      |   const = str2num(constant);
      |   name = 'CONST';
      | end;
      mask Display: fprintf('%s = %.4f',name,const);
  CONSTANT1 : Subsystem  mask(Constant){constant=TCDASD}
      mask help: Constant Block. Will dispaly constant name and value on the icon of the block
      mask init:
      | if isletter(constant(1))
      |   const = evalin('base',constant);
      |   name = constant;
      | else
      |   const = str2num(constant);
      |   name = 'CONST';
      | end;
      mask Display: fprintf('%s = %.4f',name,const);
  Multiport Switch : MultiPortSwitch  Inputs=2
  ROLAV_TC_in_DT_in : Subsystem  mask(Rolling Average - Time Constant){}
      mask help: Rolling Average - Time Constant. This filter block is the first order approximation using a time constant. Inputs include the time constant, old_ave which is the previous average value, new_value which is the new filter to filter toward, and the delta_time which is elapsed time over which to perform the filter equation.
      mask Display: fprintf('ROLAV_TC');
  dstpbr : Outport
  wires:
  iac_dlt_time/1 -> ROLAV_TC_in_DT_in/4(delta_time)
  Multiport Switch/1 -> ROLAV_TC_in_DT_in/2(Tau)
  tp/1 -> ROLAV_TC_in_DT_in/1(new_value)
  CONSTANT/1(Out) -> Multiport Switch/2
  CONSTANT1/1(Out) -> Multiport Switch/3
  ml_tc_sw/1 -> Multiport Switch/1
  ROLAV_TC_in_DT_in/1(new_ave) -> dstpbr/1  "dstpbr"
  dstpbr_in/1 -> ROLAV_TC_in_DT_in/3(old_ave)

== system mfordmodel_v1/iac_v04_001_001/normal_mode/activate_normal_mode/ipsibr_clipping ==
  trig_ipsibr_clipping : Inport
  ipsibr_kam : Inport  Port=2
  islast : Inport  Port=3
  ctptfg : Inport  Port=4
  isflag : Inport  Port=5
  iscflg : Inport  Port=6
  ml_normal_init : Inport  Port=7
  flow_running : Inport  Port=8
  pcomp_ena : Inport  Port=9
  ipsibr_clip : Subsystem  TreatAsAtomicUnit=on
  ipsibr_clipping_ctl : Stateflow chart  TreatAsAtomicUnit=on
  ipsibr : Outport
  ipsibr_fb : Outport  Port=2
  wires:
  [ipsibr_kam] -> ipsibr_clip/3(ipsibr_kam)
  ipsibr_clipping_ctl/3(ml_limit_sw) -> ipsibr_clip/4(ml_limit_sw)  "ml_limit_sw"
  [ml_normal_init] -> ipsibr_clip/5(ml_normal_init)
  ipsibr_clipping_ctl/2(ml_min_clip) -> ipsibr_clip/2(ml_min_clip)  "ml_min_clip"
  ipsibr_clipping_ctl/1(ml_max_clip) -> ipsibr_clip/1(ml_max_clip)  "ml_max_clip"
  ipsibr_clip/1(ipsibr) -> ipsibr/1
  ipsibr_clip/2(ipsibr_fb) -> ipsibr_fb/1
  [do_ipsibr_clip] -> ipsibr_clip/Trigger
  ml_normal_init/1 -> [ml_normal_init], ipsibr_clipping_ctl/5(ml_normal_init)
  ipsibr_kam/1 -> ipsibr_clipping_ctl/6(ipsibr), [ipsibr_kam]
  pcomp_ena/1 -> ipsibr_clipping_ctl/8(pcomp_ena)
  flow_running/1 -> ipsibr_clipping_ctl/7(flow_running)
  iscflg/1 -> ipsibr_clipping_ctl/4(iscflg)
  trig_ipsibr_clipping/1 -> ipsibr_clipping_ctl/Trigger
  islast/1 -> ipsibr_clipping_ctl/2(islast)
  isflag/1 -> ipsibr_clipping_ctl/1(isflag)
  ctptfg/1 -> ipsibr_clipping_ctl/3(ctptfg)
  ipsibr_clipping_ctl/4(do_ipsibr_clip()) -> [do_ipsibr_clip]  "do_ipsibr_clip"
